simulink model "Simulations_section73"  (R2023a)
settings: Solver=ode23tb  StartTime=0.0  StopTime=time_end  MaxStep=1e-3  RelTol=1e-5  EnableMultiTasking=on
values from neighbouring files (symbols this model uses):
  A = [0 1;1 1]    [Section73.m]
  Akmax = CorrM.a    [Section73.m]
  Akmin = Corrm.a    [Section73.m]
  B = [0;1]    [Section73.m]
  Bkmax = CorrM.b    [Section73.m]
  Bkmin = Corrm.b    [Section73.m]
  C = [-1 0]    [Section73.m]
  Ckmax = CorrM.c    [Section73.m]
  Ckmin = Corrm.c    [Section73.m]
  D = 0    [Section73.m]
  Dkmax = CorrM.d    [Section73.m]
  Dkmin = Corrm.d    [Section73.m]
  rhomax = rhoM    (= 0.99)    [Section73.m]
  rhomin = rhom    (= 0.1)    [Section73.m]
  scenario = input('Which scenario would you like to run: 1 or 2 ? Answer = ')    [Section73.m]
libraries: cstblocks x1, simulink x1
settings Model: Creator=senameo  LastModifiedBy=senameo
settings SolverCC: AlgebraicLoopSolver=LineSearch
settings DataIOCC: LimitDataPoints=on  SaveFormat=Array  SignalLoggingSaveFormat=ModelDataLogs  ReturnWorkspaceOutputs=off
settings OptimizationCC: InitFltsAndDblsToZero=on  LifeSpan=inf
settings DebuggingCC: SaveWithParameterizedLinksMsg=none  UnderspecifiedInitializationDetection=Classic  MergeDetectMultiDrivingBlocksExec=none  SignalResolutionControl=TryResolveAllWithWarning  SolverPrmCheckMsg=warning  MultiTaskDSMMsg=warning  MultiTaskCondExecSysMsg=none  FcnCallInpInsideContextMsg=warning  UnconnectedInputMsg=warning  UnconnectedOutputMsg=warning  UnconnectedLineMsg=warning  SFUnexpectedBacktrackingDiag=warning  SFNoUnconditionalDefaultTransitionDiag=warning  SFExecutionAtInitializationDiag=none  ArithmeticOperatorsInVariantConditions=warning
settings HardwareCC: ProdBitPerPointer=32  ProdBitPerSizeT=32  ProdBitPerPtrDiffT=32  ProdLargestAtomicFloat=None  ProdIntDivRoundTo=Undefined  ProdEndianess=Unspecified  ProdWordSize=32  ProdHWDeviceType=32-bit Generic
settings ModelReferenceCC: EnableRefExpFcnMdlSchedulingChecks=on  PropagateSignalLabelsOutOfModel=off
settings SFSimCC: CustomCodeUndefinedFunction=UseInterfaceOnly
settings RTWCC: DLArmComputeVersion=19.05
settings CodeAppCC: StateflowObjectComments=on
settings GRTTargetCC: TargetFcnLib=ansi_tfl_tmw.mat  TargetLangStandard=C89/C90 (ANSI)  CombineOutputUpdateFcns=off  GRTInterface=on
settings ConfigComp: CovMetricSettings=dw  CovSaveCumulativeToWorkspaceVar=on  CovSaveSingleToWorkspaceVar=on

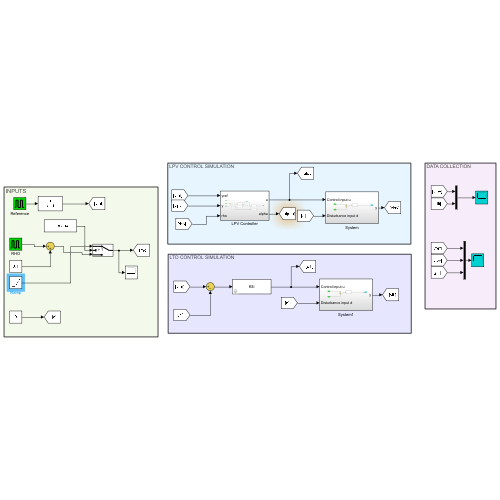
[thumbnail: Simulink's stored preview of the top-level diagram]
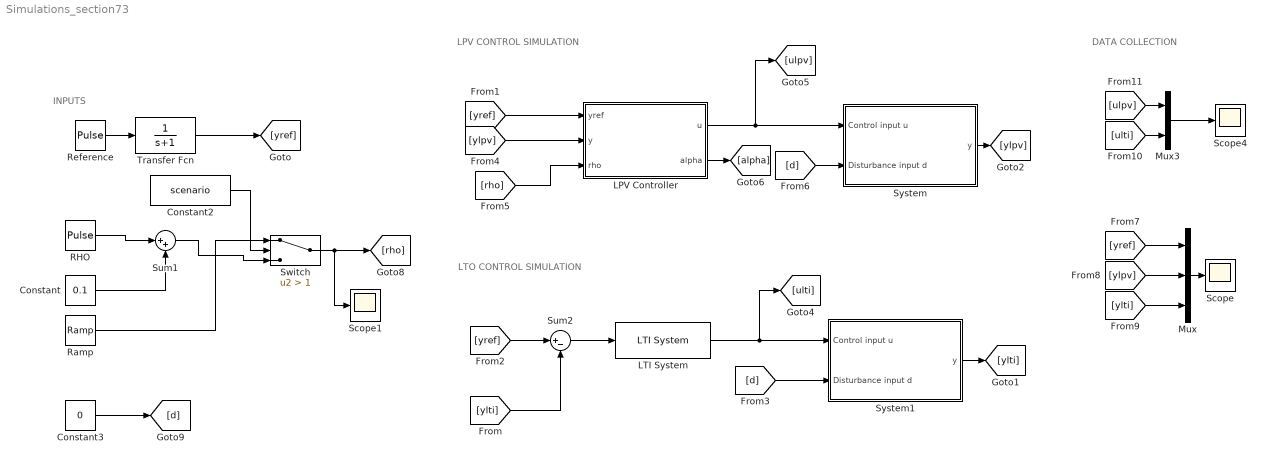
== system Simulations_section73 ==
  note: DATA COLLECTION
  note: LTO CONTROL SIMULATION
  note: LPV CONTROL SIMULATION
  note: INPUTS
  Constant : Constant  Value=0.1
  Constant2 : Constant  Value=scenario
  Constant3 : Constant  Value=0
  LPV Controller : Subsystem
  LTI System : cstblocks/LTI System  sys=Klti  IC=[]
  Mux : Mux  Inputs=3
  Mux3 : Mux  Inputs=2
  RHO : DiscretePulseGenerator  PulseType=Time based  Amplitude=0.9  Period=100  PulseWidth=50
  Ramp : simulink/Sources/Ramp  slope=-0.0015  start=0  InitialOutput=1
  Reference : DiscretePulseGenerator  PulseType=Time based  Period=50  PulseWidth=50
  Scope : Scope
  Scope1 : Scope
  Scope4 : Scope
  Sum1 : Sum  Inputs=|++  InputSameDT=on  SaturateOnIntegerOverflow=on  OutDataTypeStr=Inherit: Same as first input
  Sum2 : Sum  Inputs=|+-  InputSameDT=on  SaturateOnIntegerOverflow=on  OutDataTypeStr=Inherit: Same as first input
  Switch : Switch  Criteria=u2 > Threshold  Threshold=1  SaturateOnIntegerOverflow=off  InputSameDT=off
  System : Subsystem
  System1 : Subsystem
  Transfer Fcn : TransferFcn  Denominator=[1 1]
  wires:
  Mux/1 -> Scope/1
  Mux3/1 -> Scope4/1
  System1/1(y) -> [ylti]
  System/1(y) -> [ylpv]
  LPV Controller/1(u) -> [ulpv], System/1(Control input u)
  LTI System/1 -> [ulti], System1/1(Control input u)
  [yref] -> LPV Controller/1(yref)
  [yref] -> Sum2/1
  [ylti] -> Sum2/2
  Sum2/1 -> LTI System/1
  [d] -> System1/2(Disturbance input d)
  [ylpv] -> LPV Controller/2(y)
  [rho] -> LPV Controller/3(rho)
  LPV Controller/2(alpha) -> [alpha]
  [d] -> System/2(Disturbance input d)
  [yref] -> Mux/1
  [ylpv] -> Mux/2
  [ylti] -> Mux/3
  [ulti] -> Mux3/2
  [ulpv] -> Mux3/1
  Sum1/1 -> Switch/3
  Ramp/1 -> Switch/1
  Switch/1 -> Scope1/1, [rho]
  Constant2/1 -> Switch/2
  Constant3/1 -> [d]
  RHO/1 -> Sum1/1
  Constant/1 -> Sum1/2
  Transfer Fcn/1 -> [yref]
  Reference/1 -> Transfer Fcn/1

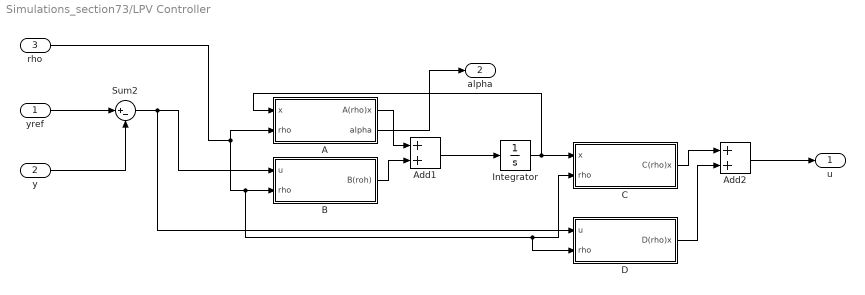
== system Simulations_section73/LPV Controller ==
  yref : Inport
  y : Inport  Port=2
  rho : Inport  Port=3
  A : Subsystem
  Add1 : Sum
  Add2 : Sum
  B : Subsystem
  C : Subsystem
  D : Subsystem
  Integrator : Integrator
  Sum2 : Sum  Inputs=|+-  InputSameDT=on  SaturateOnIntegerOverflow=on  OutDataTypeStr=Inherit: Same as first input
  u : Outport  VectorParamsAs1DForOutWhenUnconnected=off
  alpha : Outport  Port=2  VectorParamsAs1DForOutWhenUnconnected=off
  wires:
  y/1 -> Sum2/2
  Sum2/1 -> D/1(u), B/1(u)
  yref/1 -> Sum2/1
  Add2/1 -> u/1
  rho/1 -> D/2(rho), C/2(rho), B/2(rho), A/2(rho)
  A/1(A(rho)x) -> Add1/1
  B/1(B(roh)) -> Add1/2
  Add1/1 -> Integrator/1
  Integrator/1 -> A/1(x), C/1(x)
  D/1(D(rho)x) -> Add2/2
  C/1(C(rho)x) -> Add2/1
  A/2(alpha) -> alpha/1

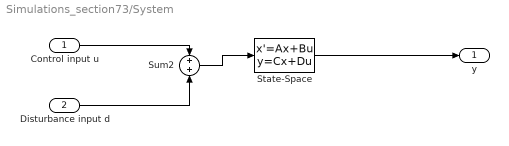
== system Simulations_section73/System ==
  Control input u : Inport
  Disturbance input d : Inport  Port=2
  State-Space : StateSpace  A=A  B=B  C=C  D=D  InitialCondition=0
  Sum2 : Sum  Inputs=+|+  InputSameDT=on  SaturateOnIntegerOverflow=on  OutDataTypeStr=Inherit: Same as first input
  y : Outport  VectorParamsAs1DForOutWhenUnconnected=off
  wires:
  Disturbance input d/1 -> Sum2/2
  State-Space/1 -> y/1
  Sum2/1 -> State-Space/1
  Control input u/1 -> Sum2/1

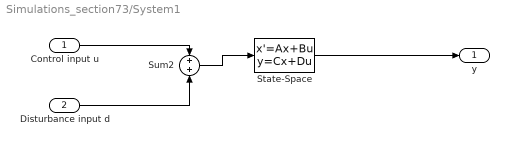
== system Simulations_section73/System1 ==
  Control input u : Inport
  Disturbance input d : Inport  Port=2
  State-Space : StateSpace  A=A  B=B  C=C  D=D  InitialCondition=0
  Sum2 : Sum  Inputs=+|+  InputSameDT=on  SaturateOnIntegerOverflow=on  OutDataTypeStr=Inherit: Same as first input
  y : Outport  VectorParamsAs1DForOutWhenUnconnected=off
  wires:
  Disturbance input d/1 -> Sum2/2
  State-Space/1 -> y/1
  Sum2/1 -> State-Space/1
  Control input u/1 -> Sum2/1

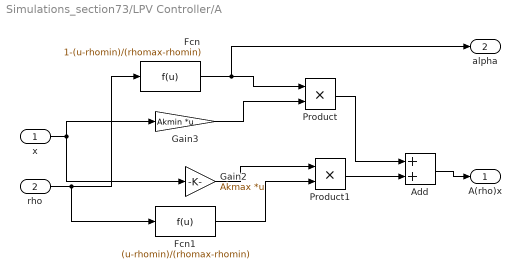
== system Simulations_section73/LPV Controller/A ==
  x : Inport
  rho : Inport  Port=2
  Add : Sum
  Fcn : Fcn  Expr=1-(u-rhomin)/(rhomax-rhomin)
  Fcn1 : Fcn  Expr=(u-rhomin)/(rhomax-rhomin)
  Gain2 : Gain  Gain=Akmax  Multiplication=Matrix(K*u)
  Gain3 : Gain  Gain=Akmin  Multiplication=Matrix(K*u)
  Product : Product
  Product1 : Product
  A(rho)x : Outport  VectorParamsAs1DForOutWhenUnconnected=off
  alpha : Outport  Port=2  VectorParamsAs1DForOutWhenUnconnected=off
  wires:
  Gain2/1 -> Product1/1
  Gain3/1 -> Product/2
  Fcn1/1 -> Product1/2
  Fcn/1 -> alpha/1, Product/1
  Add/1 -> A(rho)x/1
  Product1/1 -> Add/2
  Product/1 -> Add/1
  rho/1 -> Fcn1/1, Fcn/1
  x/1 -> Gain2/1, Gain3/1

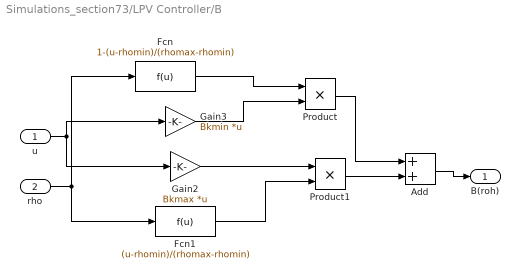
== system Simulations_section73/LPV Controller/B ==
  u : Inport
  rho : Inport  Port=2
  Add : Sum
  Fcn : Fcn  Expr=1-(u-rhomin)/(rhomax-rhomin)
  Fcn1 : Fcn  Expr=(u-rhomin)/(rhomax-rhomin)
  Gain2 : Gain  Gain=Bkmax  Multiplication=Matrix(K*u)
  Gain3 : Gain  Gain=Bkmin  Multiplication=Matrix(K*u)
  Product : Product
  Product1 : Product
  B(roh) : Outport  VectorParamsAs1DForOutWhenUnconnected=off
  wires:
  Gain2/1 -> Product1/1
  Gain3/1 -> Product/2
  Fcn1/1 -> Product1/2
  Fcn/1 -> Product/1
  Add/1 -> B(roh)/1
  Product1/1 -> Add/2
  Product/1 -> Add/1
  rho/1 -> Fcn1/1, Fcn/1
  u/1 -> Gain2/1, Gain3/1

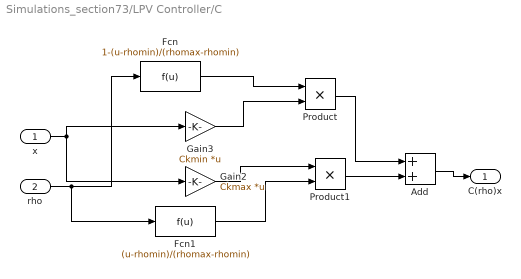
== system Simulations_section73/LPV Controller/C ==
  x : Inport
  rho : Inport  Port=2
  Add : Sum
  Fcn : Fcn  Expr=1-(u-rhomin)/(rhomax-rhomin)
  Fcn1 : Fcn  Expr=(u-rhomin)/(rhomax-rhomin)
  Gain2 : Gain  Gain=Ckmax  Multiplication=Matrix(K*u)
  Gain3 : Gain  Gain=Ckmin  Multiplication=Matrix(K*u)
  Product : Product
  Product1 : Product
  C(rho)x : Outport  VectorParamsAs1DForOutWhenUnconnected=off
  wires:
  Gain2/1 -> Product1/1
  Gain3/1 -> Product/2
  Fcn1/1 -> Product1/2
  Fcn/1 -> Product/1
  Add/1 -> C(rho)x/1
  Product1/1 -> Add/2
  Product/1 -> Add/1
  rho/1 -> Fcn1/1, Fcn/1
  x/1 -> Gain2/1, Gain3/1

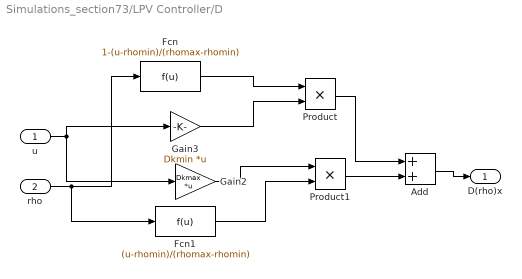
== system Simulations_section73/LPV Controller/D ==
  u : Inport
  rho : Inport  Port=2
  Add : Sum
  Fcn : Fcn  Expr=1-(u-rhomin)/(rhomax-rhomin)
  Fcn1 : Fcn  Expr=(u-rhomin)/(rhomax-rhomin)
  Gain2 : Gain  Gain=Dkmax  Multiplication=Matrix(K*u)
  Gain3 : Gain  Gain=Dkmin  Multiplication=Matrix(K*u)
  Product : Product
  Product1 : Product
  D(rho)x : Outport  VectorParamsAs1DForOutWhenUnconnected=off
  wires:
  Gain2/1 -> Product1/1
  Gain3/1 -> Product/2
  Fcn1/1 -> Product1/2
  Fcn/1 -> Product/1
  Add/1 -> D(rho)x/1
  Product1/1 -> Add/2
  Product/1 -> Add/1
  rho/1 -> Fcn1/1, Fcn/1
  u/1 -> Gain2/1, Gain3/1
